simulink model "initialloc_acc_70"  (R2025b)
settings: Solver=ode4  StartTime=t_init  StopTime=t_end  FixedStep=t_step  RelTol=1e-3
undefined symbols (not defined in the file): ai, Ai, alpha_si, As, bi, Bs, Cs, Ds, k1i, k2i, k3i, L, lambdai, loci, mi, n_modos, side, Twaitadd, v0, v0p, vi, wi, x0
settings Model: VariantFading=off  Creator=LEGION  LastModifiedBy=LEGION
settings ModelReferenceCC: EnableRefExpFcnMdlSchedulingChecks=on
settings RTWCC: GPUComputeCapability=3.5

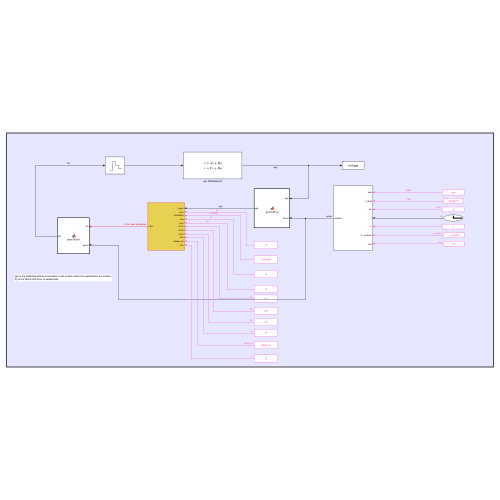
[thumbnail: Simulink's stored preview of the top-level diagram]
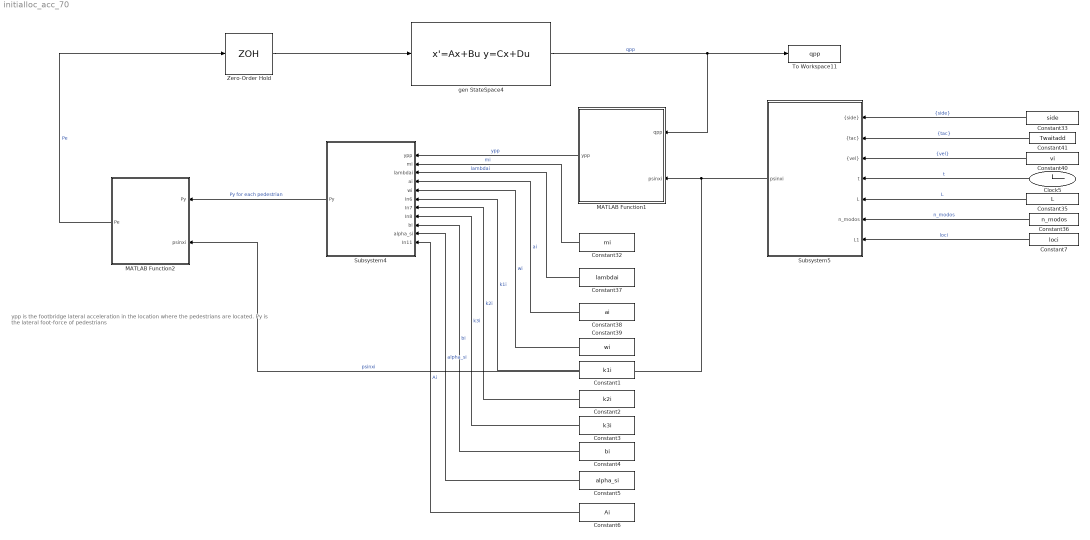
== system initialloc_acc_70 ==
  note: ypp is the footbridge lateral acceleration in the location where the pedestrians are located.
      | Py is the lateral foot-force of pedestrians
  Clock5 : Clock
  Constant1 : Constant  Value=k1i
  Constant2 : Constant  Value=k2i
  Constant3 : Constant  Value=k3i
  Constant32 : Constant  Value=mi
  Constant33 : Constant  Value=side
  Constant35 : Constant  Value=L
  Constant36 : Constant  Value=n_modos
  Constant37 : Constant  Value=lambdai
  Constant38 : Constant  Value=ai
  Constant39 : Constant  Value=wi
  Constant4 : Constant  Value=bi
  Constant40 : Constant  Value=vi
  Constant41 : Constant  Value=Twaitadd
  Constant5 : Constant  Value=alpha_si
  Constant6 : Constant  Value=Ai
  Constant7 : Constant  Value=loci
  MATLAB Function1 : MATLAB Function  TreatAsAtomicUnit=on
  MATLAB Function2 : MATLAB Function  TreatAsAtomicUnit=on
  Subsystem4 : Subsystem
  Subsystem5 : Subsystem
  To Workspace11 : ToWorkspace  VariableName=qpp  SaveFormat=Timeseries  SampleTime=-1
  Zero-Order Hold : ZeroOrderHold  SampleTime=-1
  gen StateSpace4 : StateSpace  A=As  B=Bs  C=Cs  D=Ds  InitialCondition=x0
  wires:
  gen StateSpace4/1 -> MATLAB Function1/1(qpp), To Workspace11/1  "qpp"
  MATLAB Function1/1(ypp) -> Subsystem4/1(ypp)  "ypp"
  Constant38/1 -> Subsystem4/4(ai)  "ai"
  Constant37/1 -> Subsystem4/3(lambdai)  "lambdai"
  Constant32/1 -> Subsystem4/2(mi)  "mi"
  Constant33/1 -> Subsystem5/1("{side}")  "{side}"
  Constant40/1 -> Subsystem5/3("{vel}")  "{vel}"
  Constant36/1 -> Subsystem5/6(n_modos)  "n_modos"
  Constant39/1 -> Subsystem4/5(wi)  "wi"
  Constant41/1 -> Subsystem5/2("{tac}")  "{tac}"
  MATLAB Function2/1(Pe) -> Zero-Order Hold/1  "Pe"
  Constant35/1 -> Subsystem5/5(L)  "L"
  Clock5/1 -> Subsystem5/4(t)  "t"
  Subsystem4/1(Py) -> MATLAB Function2/1(Py)  "Py for each pedestrian"
  Subsystem5/1(psinxi) -> MATLAB Function2/2(psinxi), MATLAB Function1/2(psinxi)  "psinxi"
  Constant1/1 -> Subsystem4/6(In6)  "k1i"
  Constant2/1 -> Subsystem4/7(In7)  "k2i"
  Constant3/1 -> Subsystem4/8(In8)  "k3i"
  Constant4/1 -> Subsystem4/9(bi)  "bi"
  Constant5/1 -> Subsystem4/10(alpha_si)  "alpha_si"
  Constant6/1 -> Subsystem4/11(In11)  "Ai"
  Zero-Order Hold/1 -> gen StateSpace4/1
  Constant7/1 -> Subsystem5/7(L1)  "loci"

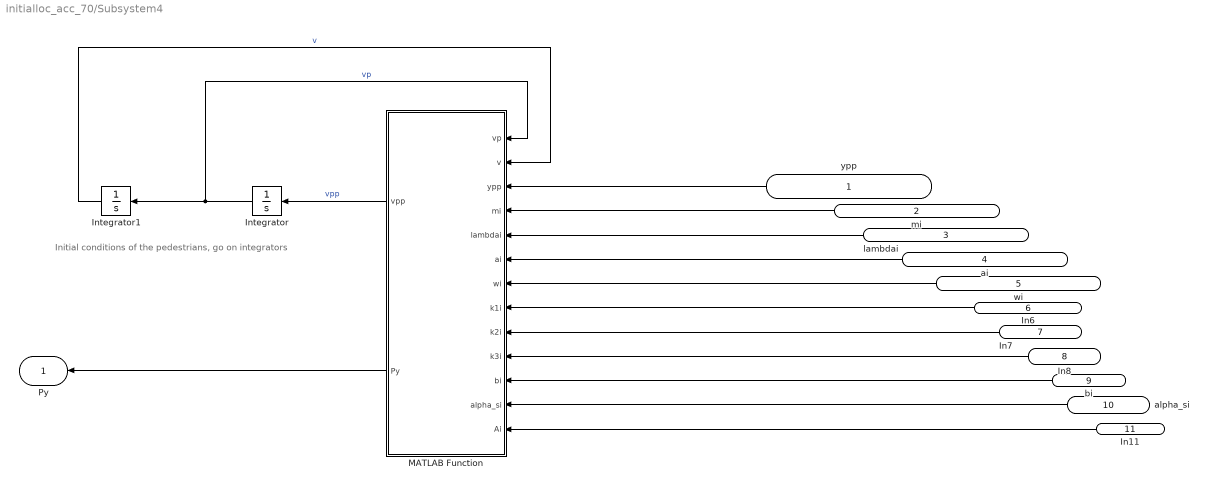
== system initialloc_acc_70/Subsystem4 ==
  note: Initial conditions of the pedestrians, go on integrators
  ypp : Inport
  mi : Inport  Port=2
  lambdai : Inport  Port=3
  ai : Inport  Port=4
  wi : Inport  Port=5
  In6 : Inport  Port=6
  In7 : Inport  Port=7
  In8 : Inport  Port=8
  bi : Inport  Port=9
  alpha_si : Inport  Port=10
  In11 : Inport  Port=11
  Integrator : Integrator  InitialCondition=v0p
  Integrator1 : Integrator  InitialCondition=v0
  MATLAB Function : MATLAB Function  TreatAsAtomicUnit=on
  Py : Outport
  wires:
  MATLAB Function/1(vpp) -> Integrator/1  "vpp"
  Integrator/1 -> MATLAB Function/1(vp), Integrator1/1  "vp"
  ypp/1 -> MATLAB Function/3(ypp)
  Integrator1/1 -> MATLAB Function/2(v)  "v"
  mi/1 -> MATLAB Function/4(mi)
  lambdai/1 -> MATLAB Function/5(lambdai)
  ai/1 -> MATLAB Function/6(ai)
  wi/1 -> MATLAB Function/7(wi)
  MATLAB Function/2(Py) -> Py/1
  In6/1 -> MATLAB Function/8(k1i)
  In7/1 -> MATLAB Function/9(k2i)
  In8/1 -> MATLAB Function/10(k3i)
  In11/1 -> MATLAB Function/13(Ai)
  bi/1 -> MATLAB Function/11(bi)
  alpha_si/1 -> MATLAB Function/12(alpha_si)

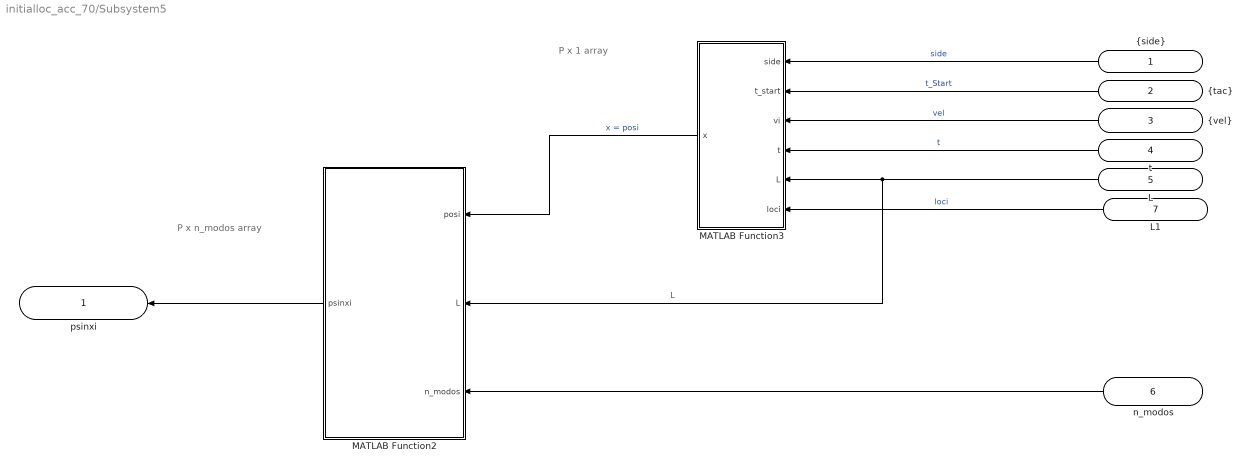
== system initialloc_acc_70/Subsystem5 ==
  note: P x 1 array
  note: P x n_modos array
  "{side}" : Inport
  "{tac}" : Inport  Port=2
  "{vel}" : Inport  Port=3
  t : Inport  Port=4
  L : Inport  Port=5
  n_modos : Inport  Port=6
  L1 : Inport  Port=7
  MATLAB Function2 : MATLAB Function  TreatAsAtomicUnit=on
  MATLAB Function3 : MATLAB Function  TreatAsAtomicUnit=on
  psinxi : Outport
  wires:
  L/1 -> MATLAB Function2/2(L), MATLAB Function3/5(L)  "L"
  MATLAB Function3/1(x) -> MATLAB Function2/1(posi)  "x = posi"
  n_modos/1 -> MATLAB Function2/3(n_modos)
  "{side}"/1 -> MATLAB Function3/1(side)  "side"
  MATLAB Function2/1(psinxi) -> psinxi/1
  "{tac}"/1 -> MATLAB Function3/2(t_start)  "t_Start"
  t/1 -> MATLAB Function3/4(t)  "t"
  "{vel}"/1 -> MATLAB Function3/3(vi)  "vel"
  L1/1 -> MATLAB Function3/6(loci)  "loci"

== matlab function initialloc_acc_70/MATLAB Function1 ==
  data: qpp input; psinxi input; ypp output
function ypp = genToPhys(qpp,psinxi)
% Generar la aceleración que expermentan todos los peatones i (desde el 1
% hasta el peatón p), sumando la respuesta modal de todos los modos (la
% contribución modal)
% ypp = sum(psinxi*qpp,2);                                                    % Sumo todas las contribuciones modales de cada modo
ypp = psinxi*qpp;

== matlab function initialloc_acc_70/MATLAB Function2 ==
  data: Py input; Pe output; psinxi input
function Pe = physToGen(Py,psinxi)
% Transforms lateral foot-forces from physical coordinates (one per pedestrian)
% to generalized coordinates (one per mode)
%
% 
%
%
Pe = psinxi.'*Py;

== matlab function initialloc_acc_70/Subsystem4/MATLAB Function ==
  data: vp input; v input; ypp input; vpp output; mi input; lambdai input; ai input; wi input; Py output; k1i input; k2i input; k3i input; bi input; alpha_si input; Ai input
function [vpp,Py] = fcn(vp, v, ypp, mi, lambdai, ai, wi, k1i, k2i, k3i, bi, alpha_si, Ai)

% Initial 
lambda1 = k1i.*lambdai./(bi.*(Ai.^2));                                      % (P x 1)
lambda2 = k2i.*lambdai.*bi./(Ai.^2);                                          % (P x 1)
lambda3 = k3i.*lambdai.*bi;                                                  % (P x 1)
% wi = wi/(2*pi)*b; % es igual a wi

% Van Der Pol Type Walker Modificado
fvdv = (lambda1.*(vp.^2) + lambda2.*(v.^2) - lambda3.*ai).*vp + (wi.^2).*v; % (P x 1)

% Aceleración del peatón
vpp = -ypp - fvdv;                                                          % (P x 1)

% Lateral foot-force applied for each pedestrian
Py = -alpha_si.*mi.*vpp;                                                    % (P x 1)

== matlab function initialloc_acc_70/Subsystem5/MATLAB Function2 ==
  data: posi input; psinxi output size=[P n_modos]; L input; n_modos input
function psinxi = psinxi(posi, L, n_modos)
% Compute psi(x) for all pedestrians
%
% psi(xi) = sin(pi*n/L*xi), where xi is the location where the i-th
% pedestrian is located in this time step
% psinxi = [ sin(1pix1/L) sin(2pix1/L) .... para todos los modos
% sin(1pix2/L) sin(2pix2/L) .... para todos los modos
% ....

% Method 1
% core_matrix = posi*(1:1:n_modos);
% M_modos = (pi/L)*core_matrix;
% psinxi = sin(M_modos);

% Method 2
psinxi = zeros(70,3);   % SPECIFY NUMBER OF PEDESTRIANS (P) AND MODES (n_modes) in zeros(P, n_modes)
for n = 1:n_modos
    psinxi(:,n) = sin(pi*n/L*posi);
end

== matlab function initialloc_acc_70/Subsystem5/MATLAB Function3 ==
  data: side input; x output; t_start input; vi input; t input; L input; loci input
function x = pedestrian_position(side, t_start, vi, t, L, loci)
% PEDESTRIAN_POSITION Determines the position of all pedestrians on the bridge.
%
% This function calculates the longitudinal position 'x' of pedestrians
% considering reflective boundaries (they turn around at 0 and L).
%
% INPUTS:
%   side    : Vector (Px1). Entry side (0: Left/Start, 1: Right/End).
%             Determines the initial walking direction.
%   t_start : Scalar. Time when the pedestrians start moving (s).
%   vi      : Vector (Px1). Walking speed (m/s).
%   t       : Scalar. Current simulation time (s).
%   L       : Scalar. Length of the bridge (m).
%   loci      : Vector (Px1). Initial position of pedestrians along the bridge (m).
%
% OUTPUTS:
%   x       : Vector (Px1). Current position of pedestrians (m).

    % 1. Determine Direction
    % Convert side (0 or 1) to a direction scalar (+1 or -1).
    % If side is 0 (Left), direction is +1. If side is 1 (Right), direction is -1.
    direction = 1 - 2 .* side; 

    % 2. Calculate Active Time
    % Calculate how long they have been walking. Result is 0 if t < t_start.
    delta_t = max(t - t_start, 0);

    % 3. Compute Virtual Position (Unbounded)
    % Equation: x_virt = x_initial + (direction * speed * time)
    x_virtual = loci + (direction .* vi .* delta_t);

    % We map the virtual position to a cycle of 2*L to simulate bouncing.
    cycle_pos = mod(x_virtual, 2*L);
    
    % Fold the domain to keep x within [0, L]
    x = min(cycle_pos, 2*L - cycle_pos);

    % If the current time t is less than t_start, force position to 0.
    if t < t_start
        x(:) = 0;
    end
